simulink model "LaneKeeping_LQR"  (R2023b)
settings: Solver=ode4  StartTime=0.0  StopTime=20  FixedStep=0.01  RelTol=1e-3
values from neighbouring files (symbols this model uses):
  A = [0,     v,      0,                          0 ... (first row only)    [lateral_lqr.m]    (also in lateral_lqr_params.mat = [0 0 0 0 15 0 0 0 0 0 -6.77248677249 0.742028985507 ... (16 )
  B = [0 ... (first row only)    [lateral_lqr.m]    (also in lateral_lqr_params.mat = [0 0 50.7936507937 33.3913043478])
  delta_max = 0.5    [lateral_lqr.m]    (also in lateral_lqr_params.mat)
  e_0 = 0.5    [lateral_lqr.m]    (also in lateral_lqr_params.mat)
  K_lqr = [3.16227766017 11.5819754962 0.102560918061 0.957809090599]    [lateral_lqr_params.mat]
  psi_0 = 0.05    [lateral_lqr.m]    (also in lateral_lqr_params.mat)
  r_0 = 0    [lateral_lqr.m]    (also in lateral_lqr_params.mat)
  vy_0 = 0    [lateral_lqr.m]    (also in lateral_lqr_params.mat)
settings Model: Creator=kblaw  LastModifiedBy=kblaw

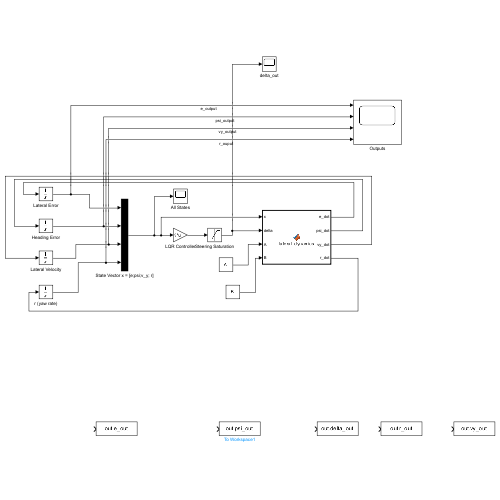
[thumbnail: Simulink's stored preview of the top-level diagram]
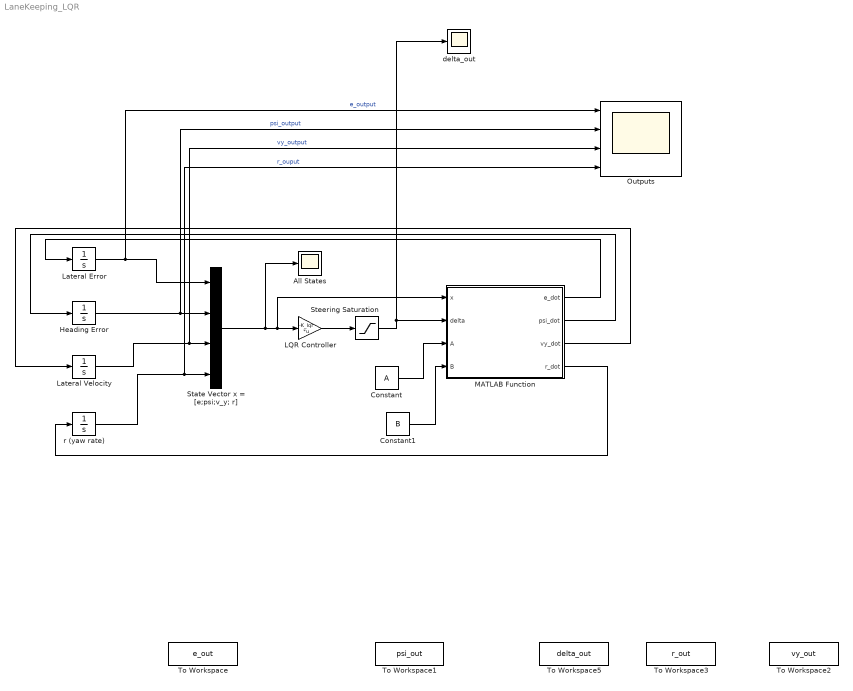
== system LaneKeeping_LQR ==
  All States : Scope
  Constant : Constant  Value=A  SampleTime=-1
  Constant1 : Constant  Value=B  SampleTime=-1
  Heading Error : Integrator  InitialCondition=psi_0
  LQR Controller : Gain  Gain=-K_lqr  Multiplication=Matrix(K*u)
  Lateral Error : Integrator  InitialCondition=e_0
  Lateral Velocity : Integrator  InitialCondition=vy_0
  MATLAB Function : MATLAB Function  TreatAsAtomicUnit=on
  Outputs : Scope  NumInputPorts=4
  State Vector x = [e;psi;v_y; r] : Mux
  Steering Saturation : Saturate  UpperLimit=delta_max  LowerLimit=-delta_max
  To Workspace : ToWorkspace  VariableName=e_out  SaveFormat=Structure With Time  SampleTime=-1
  To Workspace1 : ToWorkspace  VariableName=psi_out  SaveFormat=Structure  SampleTime=-1
  To Workspace2 : ToWorkspace  VariableName=vy_out  SaveFormat=Structure With Time  SampleTime=-1
  To Workspace3 : ToWorkspace  VariableName=r_out  SaveFormat=Structure With Time  SampleTime=-1
  To Workspace5 : ToWorkspace  VariableName=delta_out  SaveFormat=Structure With Time  SampleTime=-1
  delta_out : Scope
  r (yaw rate) : Integrator  InitialCondition=r_0
  wires:
  Lateral Error/1 -> Outputs/1, State Vector x = [e;psi;v_y; r]/1  "e_output"
  r (yaw rate)/1 -> Outputs/4, State Vector x = [e;psi;v_y; r]/4  "r_ouput"
  State Vector x = [e;psi;v_y; r]/1 -> All States/1, MATLAB Function/1(x), LQR Controller/1
  LQR Controller/1 -> Steering Saturation/1
  Steering Saturation/1 -> MATLAB Function/2(delta), delta_out/1
  MATLAB Function/1(e_dot) -> Lateral Error/1
  MATLAB Function/4(r_dot) -> r (yaw rate)/1
  Heading Error/1 -> Outputs/2, State Vector x = [e;psi;v_y; r]/2  "psi_output"
  Lateral Velocity/1 -> Outputs/3, State Vector x = [e;psi;v_y; r]/3  "vy_output"
  MATLAB Function/2(psi_dot) -> Heading Error/1
  MATLAB Function/3(vy_dot) -> Lateral Velocity/1
  Constant/1 -> MATLAB Function/3(A)
  Constant1/1 -> MATLAB Function/4(B)

== matlab function LaneKeeping_LQR/MATLAB Function ==
  data: x input; e_dot output; delta input; A input; B input; psi_dot output; vy_dot output; r_dot output
function [e_dot, psi_dot, vy_dot, r_dot] = lateral_dynamics(x, delta, A, B)
%#codegen
% Lateral vehicle dynamics: state derivatives
% Inputs:
%   x: state vector [4x1] = [e; psi; v_y; r]
%   delta: steering angle (scalar)
%   A: system matrix [4x4]
%   B: input matrix [4x1]
% Outputs:
%   e_dot, psi_dot, vy_dot, r_dot: state derivatives

% Compute state derivatives: x_dot = A*x + B*delta
x_dot = A * x + B * delta;

% Extract individual derivatives
e_dot = x_dot(1);      % lateral error rate
psi_dot = x_dot(2);    % heading error rate
vy_dot = x_dot(3);     % lateral velocity rate
r_dot = x_dot(4);      % yaw rate derivative
